simulink model "plantaOpenLoop"  (R2020b)
settings: Solver=VariableStepAuto  StartTime=0.0  StopTime=50  MaxStep=0.01  RelTol=1e-3
undefined symbols (not defined in the file): d1, d2, DZ, I, km, MAX_PWM, miu, theta0, wb, wcp, wm
settings Model: Creator=felip  LastModifiedBy=felip
settings DebuggingCC: UnconnectedInputMsg=none  UnconnectedOutputMsg=none  UnconnectedLineMsg=none  SFMachineParentedDataDiag=error
settings ModelReferenceCC: EnableRefExpFcnMdlSchedulingChecks=off

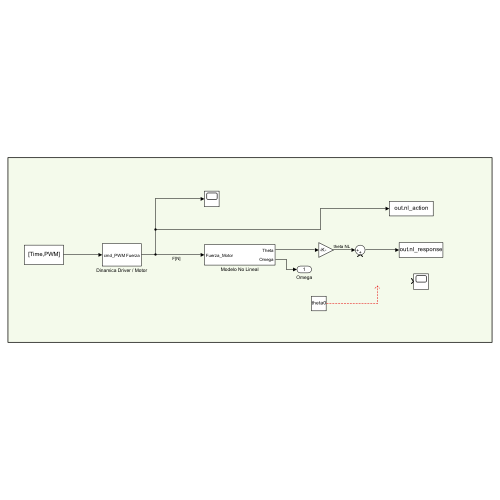
[thumbnail: Simulink's stored preview of the top-level diagram]
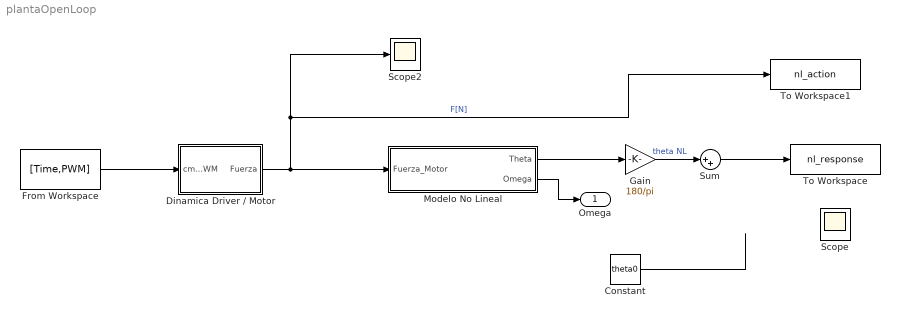
== system plantaOpenLoop ==
  Constant : Constant  Value=theta0
  Dinamica Driver / Motor : Subsystem
  From Workspace : FromWorkspace  VariableName=[Time,PWM]  SampleTime=2.5e-3
  Gain : Gain  Gain=180/pi
  Modelo No Lineal : Subsystem
  Scope : Scope
  Scope2 : Scope
  Sum : Sum  Inputs=|++
  To Workspace : ToWorkspace  VariableName=nl_response  SaveFormat=Timeseries  SampleTime=-1
  To Workspace1 : ToWorkspace  VariableName=nl_action  SaveFormat=Timeseries  SampleTime=-1
  Omega : Outport
  wires:
  Dinamica Driver / Motor/1(Fuerza) -> Scope2/1, To Workspace1/1, Modelo No Lineal/1(Fuerza_Motor)  "F[N]"
  Modelo No Lineal/1(Theta) -> Gain/1
  Modelo No Lineal/2(Omega) -> Omega/1
  From Workspace/1 -> Dinamica Driver / Motor/1(cmd_PWM)
  Gain/1 -> Sum/1  "theta NL"
  Constant/1 -> ?
  Sum/1 -> To Workspace/1

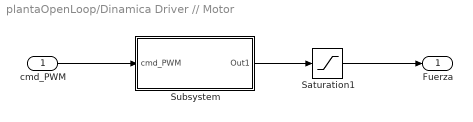
== system plantaOpenLoop/Dinamica Driver // Motor ==
  cmd_PWM : Inport
  Saturation1 : Saturate  UpperLimit=MAX_PWM
  Subsystem : Subsystem
  Fuerza : Outport
  wires:
  Saturation1/1 -> Fuerza/1
  cmd_PWM/1 -> Subsystem/1(cmd_PWM)
  Subsystem/1(Out1) -> Saturation1/1

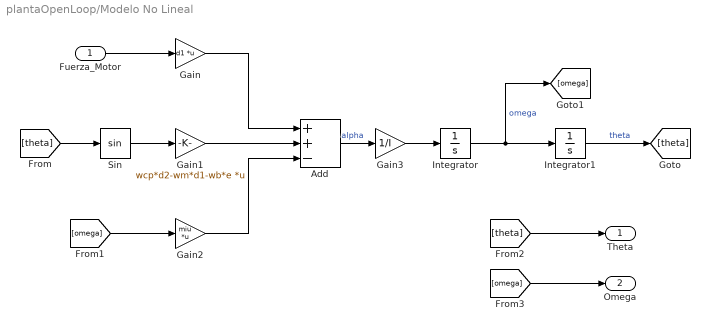
== system plantaOpenLoop/Modelo No Lineal ==
  Fuerza_Motor : Inport
  Add : Sum  Inputs=++-
  Gain : Gain  Gain=d1  Multiplication=Matrix(K*u)
  Gain1 : Gain  Gain=wcp*d2-wm*d1-wb*e  Multiplication=Matrix(K*u)
  Gain2 : Gain  Gain=miu  Multiplication=Matrix(K*u)
  Gain3 : Gain  Gain=1/I
  Integrator : Integrator
  Integrator1 : Integrator
  Sin : Trigonometry
  Theta : Outport
  Omega : Outport  Port=2
  wires:
  [omega] -> Omega/1
  Gain1/1 -> Add/2
  Integrator/1 -> [omega], Integrator1/1  "omega"
  Fuerza_Motor/1 -> Gain/1
  Integrator1/1 -> [theta]  "theta"
  Gain2/1 -> Add/3
  Gain/1 -> Add/1
  Add/1 -> Gain3/1  "alpha"
  [theta] -> Sin/1
  [omega] -> Gain2/1
  [theta] -> Theta/1
  Sin/1 -> Gain1/1
  Gain3/1 -> Integrator/1

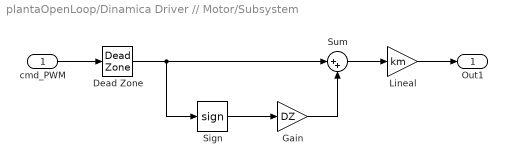
== system plantaOpenLoop/Dinamica Driver // Motor/Subsystem ==
  cmd_PWM : Inport
  Dead Zone : DeadZone  LowerValue=-DZ  UpperValue=DZ  SaturateOnIntegerOverflow=on
  Gain : Gain  Gain=DZ
  Lineal : Gain  Gain=km
  Sign : Signum
  Sum : Sum  Inputs=|++
  Out1 : Outport
  wires:
  cmd_PWM/1 -> Dead Zone/1
  Dead Zone/1 -> Sum/1, Sign/1
  Sum/1 -> Lineal/1
  Sign/1 -> Gain/1
  Gain/1 -> Sum/2
  Lineal/1 -> Out1/1
